simulink model "SimulazioneCompensatore1"  (R2019b)
settings: Solver=VariableStepAuto  StartTime=0.0  StopTime=20  RelTol=1e-3
values from neighbouring files (symbols this model uses):
  A = [0 0 1 0;0 0 0 1;-k/m1 k/m1 -c/m1 c/m1;k/m2 -k/m2 c/m2 -c/m2]    [ValoriCaso1.m]    (also in ValoriCaso2.m; ValoriParametri.m; ValoriParametri1.m; ValoriParametri2.m)
  B = [0;0;1/m1;0]    [ValoriCaso1.m]    (also in ValoriCaso2.m; ValoriParametri.m; ValoriParametri1.m; ValoriParametri2.m)
  C = [1 0 0 0]    [ValoriCaso1.m]    (also in ValoriCaso2.m; ValoriParametri.m; ValoriParametri1.m; ValoriParametri2.m)
  D = 0    [ValoriCaso1.m]    (also in ValoriCaso2.m; ValoriParametri1.m; ValoriParametri2.m)
  x0 = [0;5;0;0]    [ValoriParametri.m]    (also in ValoriParametri1.m; ValoriParametri2.m)
settings Model: Creator=sugam  LastModifiedBy=sugam

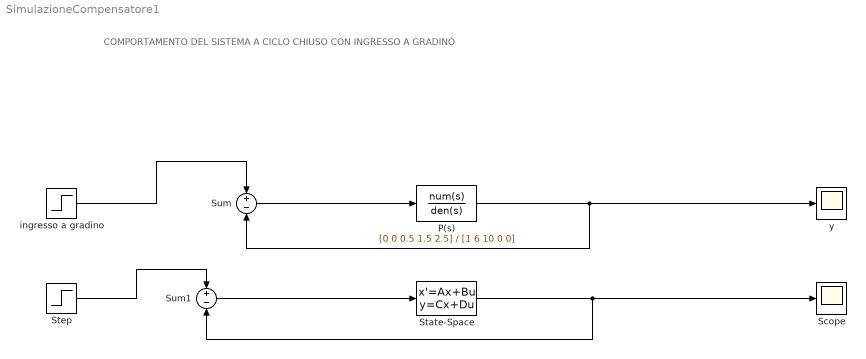
== system SimulazioneCompensatore1 ==
  note: COMPORTAMENTO DEL SISTEMA A CICLO CHIUSO CON INGRESSO A GRADINO
  P(s) : TransferFcn  Numerator=[0 0 0.5 1.5 2.5]  Denominator=[1 6 10 0 0]
  Scope : Scope
  State-Space : StateSpace  A=A  B=B  C=C  D=D  InitialCondition=x0
  Step : Step  Time=0  SampleTime=0
  Sum : Sum  Inputs=+-
  Sum1 : Sum  Inputs=+-
  ingresso a gradino : Step  Time=0  SampleTime=0
  y : Scope
  wires:
  P(s)/1 -> y/1, Sum/2
  State-Space/1 -> Sum1/2, Scope/1
  Sum/1 -> P(s)/1
  ingresso a gradino/1 -> Sum/1
  Sum1/1 -> State-Space/1
  Step/1 -> Sum1/1
